simulink model "DP2_simlink"  (R2024b)
settings: Solver=FixedStepDiscrete  StartTime=0.0  StopTime=200  FixedStep=10  RelTol=1e-3
values from neighbouring files (symbols this model uses):
  A = [0,                           1,                           0,                           0,                           0,                           0 ... (first row only)    [DP2.m]
  Ad = sys_d.A    [DP2.m]
  Bd = sys_d.B    [DP2.m]
  Cd = sys_d.C    [DP2.m]
  Dd = sys_d.D    [DP2.m]
  Q = diag([1/phi_max^2,  1/rate_max^2,            1/phi_max^2,  1/rate_max^2,            1/phi_max^2,  1/rate_max^2])    [lqr_controller.m]
  R_inv = diag(1./diag(R))    [lqr_controller.m]
undefined symbols (not defined in the file or in its folder): P0
settings Model: Creator=zalak  LastModifiedBy=zalak

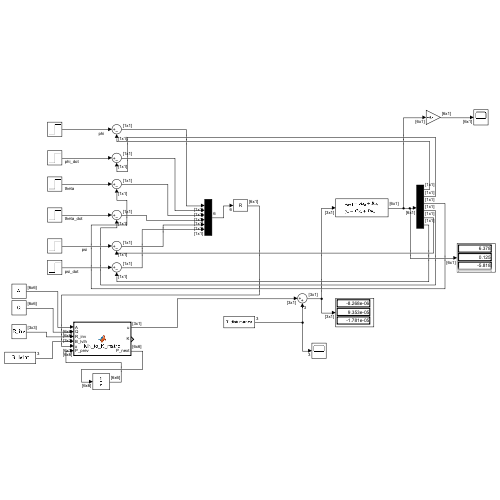
[thumbnail: Simulink's stored preview of the top-level diagram]
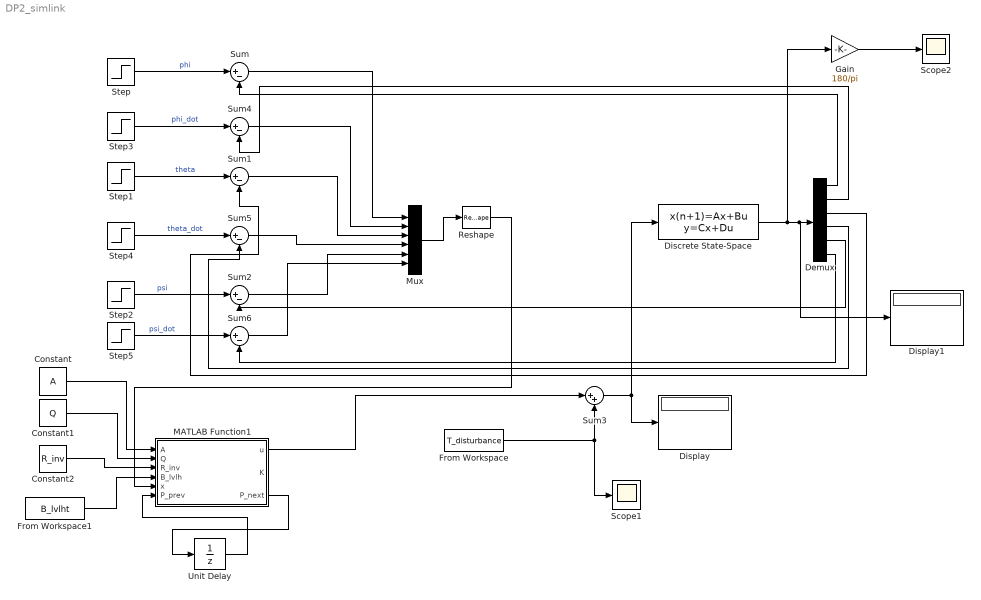
== system DP2_simlink ==
  Constant : Constant  Value=A
  Constant1 : Constant  Value=Q
  Constant2 : Constant  Value=R_inv
  Demux : Demux  Outputs=6
  Discrete State-Space : DiscreteStateSpace  A=Ad  B=Bd  C=Cd  D=Dd  InitialCondition=[pi/3, 0, pi/3, 0, pi/3, 0]  SampleTime=10
  Display : Display
  Display1 : Display
  From Workspace : FromWorkspace  VariableName=T_disturbance
  From Workspace1 : FromWorkspace  VariableName=B_lvlht  SampleTime=10
  Gain : Gain  Gain=180/pi
  MATLAB Function1 : MATLAB Function  TreatAsAtomicUnit=on
  Mux : Mux  Inputs=6
  Reshape : Reshape  OutputDimensionality=Customize  OutputDimensions=[6,1]
  Scope1 : Scope
  Scope2 : Scope
  Step{,1..5} (6 alike) : Step  Time=0  After=0  SampleTime=10
  Sum{,1..2,4..6} (6 alike) : Sum  Inputs=|+-
  Sum3 : Sum  Inputs=|++
  Unit Delay : UnitDelay  InitialCondition=P0  SampleTime=10  HasFrameUpgradeWarning=on
  wires:
  Demux/1 -> Sum/2
  Step/1 -> Sum/1  "phi"
  Step2/1 -> Sum2/1  "psi"
  Sum/1 -> Mux/1
  Sum1/1 -> Mux/3
  Step1/1 -> Sum1/1  "theta"
  Sum2/1 -> Mux/5
  Mux/1 -> Reshape/1
  Reshape/1 -> MATLAB Function1/5(x)
  MATLAB Function1/1(u) -> Sum3/1
  Sum3/1 -> Display/1, Discrete State-Space/1
  From Workspace/1 -> Scope1/1, Sum3/2
  Gain/1 -> Scope2/1
  From Workspace1/1 -> MATLAB Function1/4(B_lvlh)
  Constant/1 -> MATLAB Function1/1(A)
  Constant1/1 -> MATLAB Function1/2(Q)
  Constant2/1 -> MATLAB Function1/3(R_inv)
  MATLAB Function1/3(P_next) -> Unit Delay/1
  Unit Delay/1 -> MATLAB Function1/6(P_prev)
  Discrete State-Space/1 -> Gain/1, Display1/1, Demux/1
  Step3/1 -> Sum4/1  "phi_dot"
  Demux/3 -> Sum1/2
  Demux/5 -> Sum2/2
  Demux/2 -> Sum4/2
  Sum4/1 -> Mux/2
  Step4/1 -> Sum5/1  "theta_dot"
  Demux/4 -> Sum5/2
  Sum5/1 -> Mux/4
  Sum6/1 -> Mux/6
  Demux/6 -> Sum6/2
  Step5/1 -> Sum6/1  "psi_dot"

== matlab function DP2_simlink/MATLAB Function1 ==
  data: A input; Q input; R_inv input; B_lvlh input; x input; u output; K output; P_next output; P_prev input
function [u, K, P_next] = lvlh_to_K_matrix(A, Q, R_inv, B_lvlh, x, P_prev)
%% Step 1: LVLH to body (from attitude state, small angle ok near nominal)
phi = x(1); theta = x(3); psi = x(5);

% GOOSE 2U inertia  [kg·m²]
Ix = 0.00333;
Iy = 0.01020;
Iz = 0.01020;
dt = 10;
 
% SSO orbital rate at 515 km  [rad/s]
omega = 2*pi / 5695.5;

Rx = [1,      0,       0;
      0,  cos(phi), sin(phi);
      0, -sin(phi), cos(phi)];

Ry = [cos(theta), 0, -sin(theta);
      0,          1,  0;
      sin(theta), 0,  cos(theta)];

Rz = [cos(psi),  sin(psi), 0;
     -sin(psi),  cos(psi), 0;
      0,         0,        1];

R_lvlh2body = Rz * Ry * Rx;
B_body = R_lvlh2body * B_lvlh;

Bx = B_body(1);
By = B_body(2);
Bz = B_body(3);
 
B_cross = [  0,   Bz,  -By;
            -Bz,   0,   Bx;
             By,  -Bx,   0 ];
 
B_tv = zeros(6, 3);
B_tv(2, :) = B_cross(1, :) / Ix;   % phi_dot   driven by row 1 of B_cross
B_tv(4, :) = B_cross(3, :) / Iz;   % theta_dot driven by row 3 of B_cross
B_tv(6, :) = B_cross(2, :) / Iy;   % psi_dot   driven by row 2 of B_cross
 
%% ── Step 2: Differential Riccati Equation RHS ────────────────────────────
% dP/dt = A'P + PA - P B(t) R⁻¹ B(t)' P + Q
%
% All terms computed explicitly so the Simulink code generation path
% sees only basic matrix operations — no lqr(), no ode45().

P = P_prev;
P = (P + P') / 2;          % enforce symmetry — kills floating-point drift
 
AtP      = A'  * P;
PA_term  = P   * A;
PB       = P   * B_tv;                   % 6×3
PBRiBtP  = PB  * R_inv * (B_tv' * P);   % 6×6  = PB · R⁻¹ · B'P
 
dP = AtP + PA_term - PBRiBtP + Q;       % 6×6
 
%% ── Step 3: Forward Euler integration ───────────────────────────────────
% P(k+1) = P(k) + dt * dP/dt
%
% Forward Euler is deliberately chosen here over RK4 because:
%   a) the control period (100ms) is much shorter than the Riccati
%      time constant (many orbital periods), so the error is negligible;
%   b) it maps to a single multiply-add on the STM32 with no sub-steps,
%      which is exactly what you want when porting this firmware.
 
P_next = P + dt * dP;
P_next = (P_next + P_next') / 2;        % re-symmetrise after integration
 
%% ── Step 4: Instantaneous gain  K = R⁻¹ B(t)' P(t+dt) ──────────────────
% Use the *updated* P so K is consistent with the next state, not the
% current one — this is the standard receding-horizon convention.
 
K = R_inv * (B_tv' * P_next);           % 3×6
 
%% ── Step 5: Control law with saturation ─────────────────────────────────
u = -K * x;                         % 3×1  [N·m]
% 
% u = max(-tau_max, min(tau_max, u_raw)); % element-wise saturation

end
